simulink model "PD_Model"  (R2015b)
settings: Solver=VariableStepAuto  StartTime=0.0  StopTime=10  RelTol=1e-3
values from neighbouring files (symbols this model uses):
  C = 1E-6    (= 1e-06)    [PD_Model_script.m]    (also in PD_TF_Model.m)
  C0 = 10E-9    (= 1e-08)    [PD_Model_script.m]
  R = 100E+6    (= 100000000)    [PD_Model_script.m]    (also in PD_TF_Model.m = 100)
  R0 = 1E+9    (= 1000000000)    [PD_Model_script.m]
  S = 1    [PD_Model_script.m]
  v0 = 0    [PD_Model_script.m]    (also in PD_TF_Model.m = 100000)
  w0 = 10    [PD_Model_script.m]    (also in PD_TF_Model.m)
settings Model: Creator=lukaskiechle  LastModifiedBy=lukaskiechle

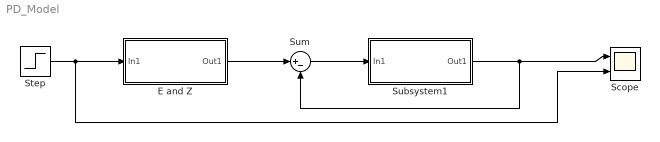
== system PD_Model ==
  E and Z : Subsystem
  Scope : Scope  NumInputPorts=2
  Step : Step  SampleTime=0
  Subsystem1 : Subsystem
  Sum : Sum  Inputs=|+-
  wires:
  E and Z/1(Out1) -> Sum/1
  Sum/1 -> Subsystem1/1(In1)
  Subsystem1/1(Out1) -> Sum/2, Scope/1
  Step/1 -> Scope/2, E and Z/1(In1)

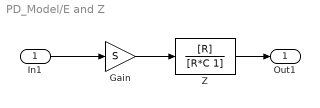
== system PD_Model/E and Z ==
  In1 : Inport
  Gain : Gain  Gain=S
  Z : TransferFcn  Numerator=[R]  Denominator=[R*C 1]
  Out1 : Outport
  wires:
  Gain/1 -> Z/1
  Z/1 -> Out1/1
  In1/1 -> Gain/1

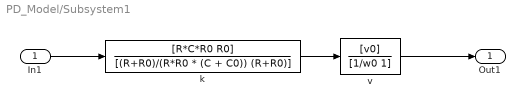
== system PD_Model/Subsystem1 ==
  In1 : Inport
  k : TransferFcn  Numerator=[R*C*R0 R0]  Denominator=[(R+R0)/(R*R0 * (C + C0)) (R+R0)]
  v : TransferFcn  Numerator=[v0]  Denominator=[1/w0 1]
  Out1 : Outport
  wires:
  v/1 -> Out1/1
  k/1 -> v/1
  In1/1 -> k/1
